simulink model "Q1_Part_d"  (R2015a)
settings: Solver=ode45  StartTime=0.0  StopTime=180  RelTol=1e-10  AbsTol=1e-10
libraries: cstblocks x3
settings Model: Creator=yarde_000  LastModifiedBy=yarde_000

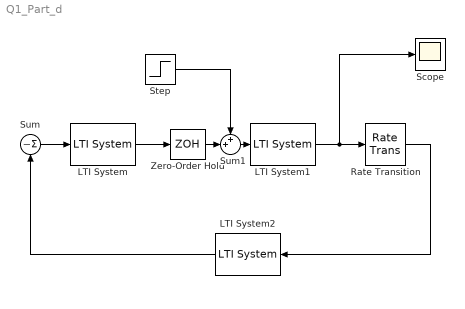
== system Q1_Part_d ==
  LTI System : cstblocks/LTI System  sys=Cd  IC=[]
  LTI System1 : cstblocks/LTI System  sys=P  IC=[]
  LTI System2 : cstblocks/LTI System  sys=F  IC=[]
  Rate Transition : RateTransition  OutPortSampleTime=ts_s
  Scope : Scope
      settings: YMin=-0.12455  YMax=1.12097  SaveName=Output
  Step : Step  Time=0  SampleTime=0
  Sum : Sum  Inputs=||-
  Sum1 : Sum  Inputs=++|
  Zero-Order Hold : ZeroOrderHold  SampleTime=-1
  wires:
  LTI System/1 -> Zero-Order Hold/1
  LTI System1/1 -> Scope/1, Rate Transition/1
  Rate Transition/1 -> LTI System2/1
  Sum/1 -> LTI System/1
  Zero-Order Hold/1 -> Sum1/2
  Sum1/1 -> LTI System1/1
  Step/1 -> Sum1/1
  LTI System2/1 -> Sum/1
